simulink library "Lib_Cntrl_LimitSelect_TMATS"  (R2019b)
settings: Solver=ode45  StartTime=0.0  StopTime=10.0  RelTol=1e-3  EnableMultiTasking=on
Description:
  | Thomas Modules
settings Model: Creator=jwchapm2  LastModifiedBy=bhisma
settings DataIOCC: LimitDataPoints=on  SaveFormat=Array  ReturnWorkspaceOutputs=off
settings OptimizationCC: ExpressionDepthLimit=2147483647  LifeSpan=inf
settings DebuggingCC: UnderspecifiedInitializationDetection=Classic  MergeDetectMultiDrivingBlocksExec=none  SolverPrmCheckMsg=warning  StateNameClashWarn=warning  SFUnexpectedBacktrackingDiag=warning  SFNoUnconditionalDefaultTransitionDiag=warning  SFExecutionAtInitializationDiag=none  ArithmeticOperatorsInVariantConditions=warning
settings HardwareCC: ProdBitPerPointer=32  ProdBitPerSizeT=32  ProdBitPerPtrDiffT=32  ProdLargestAtomicFloat=None  ProdIntDivRoundTo=Undefined  ProdEndianess=Unspecified  ProdWordSize=32  ProdHWDeviceType=32-bit Generic
settings ModelReferenceCC: PropagateSignalLabelsOutOfModel=off
settings SFSimCC: SimUseLocalCustomCode=off  CustomCodeUndefinedFunction=UseInterfaceOnly
settings RTWCC: RTWUseLocalCustomCode=off
settings CodeAppCC: StateflowObjectComments=on
settings GRTTargetCC: TargetLangStandard=C89/C90 (ANSI)  GeneratePreprocessorConditionals=Disable all
settings ConfigComp: CovMetricSettings=dw  CovHtmlReporting=on  CovSaveCumulativeToWorkspaceVar=on  CovSaveSingleToWorkspaceVar=on  CovExternalEMLEnable=off

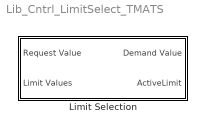
== system Lib_Cntrl_LimitSelect_TMATS ==
  Limit Selection : Subsystem  mask(T-MATS: Limit Selector){SelectVec_M=[1 1 1 -1 -1], LimitsEn_M=[1 1 1 1 1]}
      mask prompts: SelectVec_M "SelectVec_M - Selection Vector, 1, for topping limit, -1, for bottoming limit (1xn)"; LimitsEn_M "LimitsEn_M - Enable Limits: 1-Limit enabled, 0-Limit Disabled (1xn)"
      mask help: This block uses limit inputs to adjust a requested effector value. An input vector is created with a 1 for topping limits or -1 for bottom limits. The length of SelectVec_M should be equal to the length of the input vector Limit Values.
      mask init:
      | if min(abs(SelectVec_M) == 1) == 0
      |     disp('SelectVec_M in Limit Select block is improprly defined')
      | end
      mask Help: web(which('Control_TMATS_LimSel.html'),'-helpbrowser')

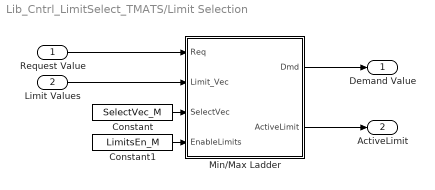
== system Lib_Cntrl_LimitSelect_TMATS/Limit Selection ==
  Request Value : Inport
  Limit Values : Inport  Port=2
  Constant : Constant  Value=SelectVec_M
  Constant1 : Constant  Value=LimitsEn_M
  Min/Max Ladder : MATLAB Function  TreatAsAtomicUnit=on
  Demand Value : Outport
  ActiveLimit : Outport  Port=2
  wires:
  Limit Values/1 -> Min/Max Ladder/2(Limit_Vec)
  Request Value/1 -> Min/Max Ladder/1(Req)
  Min/Max Ladder/1(Dmd) -> Demand Value/1
  Min/Max Ladder/2(ActiveLimit) -> ActiveLimit/1
  Constant/1 -> Min/Max Ladder/3(SelectVec)
  Constant1/1 -> Min/Max Ladder/4(EnableLimits)

== matlab function Lib_Cntrl_LimitSelect_TMATS/Limit Selection/Min//Max Ladder ==
  data: Req input; Dmd output; Limit_Vec input; SelectVec input; ActiveLimit output; EnableLimits input
function [Dmd, ActiveLimit] = fcn(Req, Limit_Vec,SelectVec, EnableLimits)
%#codegen
CurrentValue = Req;
ActiveLimit  = 0;
for i = 1:length(Limit_Vec)
    if EnableLimits(i) > 0.5
        switch SelectVec(i)
            case 1
                if CurrentValue > Limit_Vec(i)
                    CurrentValue = Limit_Vec(i);
                    ActiveLimit = i;
                end
            case -1
                if CurrentValue < Limit_Vec(i)
                    CurrentValue = Limit_Vec(i);
                    ActiveLimit = i;
                end
        end
        
    end
end


Dmd = CurrentValue;
